simulink model "ElectricalHeat"  (R2023b)
settings: Solver=VariableStepAuto  StartTime=0.0  StopTime=10  RelTol=1e-3
undefined symbols (not defined in the file): V
settings Model: ExtModeTrigDuration=100  Creator=20181234  LastModifiedBy=20181234
settings DataIOCC: StateSaveName=tmp_raccel_xout
settings OptimizationCC: EfficientMapNaN2IntZero=off
settings DebuggingCC: ModelReferenceSymbolNameMessage=none
settings HardwareCC: TargetBitPerPointer=64  TargetBitPerSizeT=64  TargetBitPerPtrDiffT=64  TargetLongLongMode=on  TargetIntDivRoundTo=Zero  TargetEndianess=LittleEndian  TargetWordSize=64  TargetHWDeviceType=MATLAB Host  ProdEqTarget=off
settings RTWCC: SystemTargetFile=raccel.tlc  TemplateMakefile=raccel_default_tmf  RTWVerbose=off  RTWUseSimCustomCode=on  CustomBLASCallback=coder.internal.blas.MATLABBLASCallback
settings CodeAppCC: GenerateComments=off  MaxIdLength=128  MangleLength=10  SimulinkBlockComments=off
settings RaccelTargetCC: TargetLangStandard=C99 (ISO)  OptimizeReductions=off  ENABLE_SLEXEC_SSBRIDGE=1  RTWCAPIParams=on  RTWCAPIRootIO=on

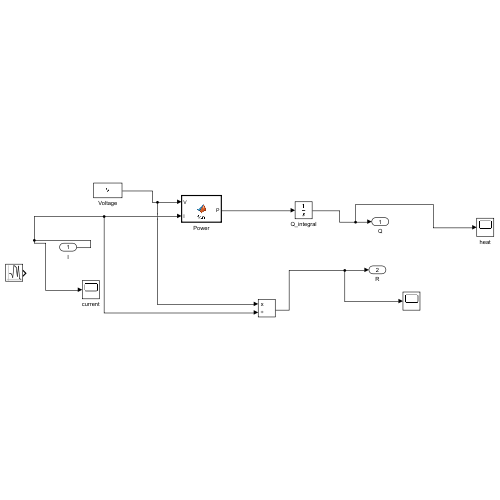
[thumbnail: Simulink's stored preview of the top-level diagram]
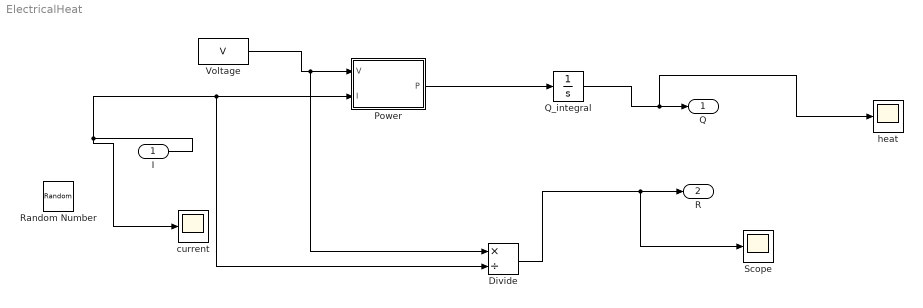
== system ElectricalHeat ==
  I : Inport
  Divide : Product  Inputs=*/
  Power : MATLAB Function  TreatAsAtomicUnit=on
  Q_integral : Integrator
  Random Number : RandomNumber  Mean=3  Variance=0.5  Seed=2569  SampleTime=1
  Scope : Scope
  Voltage : Constant  Value=V
  current : Scope
  heat : Scope
  Q : Outport
  R : Outport  Port=2
  wires:
  Voltage/1 -> Divide/1, Power/1(V)
  Power/1(P) -> Q_integral/1
  Q_integral/1 -> heat/1, Q/1
  I/1 -> current/1, Divide/2, Power/2(I)
  Divide/1 -> Scope/1, R/1

== matlab function ElectricalHeat/Power ==
  data: V input; P output; I input
function P = fcn(V,I)

P = V * I;
